simulink model "PID_dktocdo"  (Simulink 7.9)
settings: Solver=ode45  StartTime=0.0  StopTime=5  RelTol=1e-3
settings Model: Creator=Vaio  LastModifiedBy=Vaio

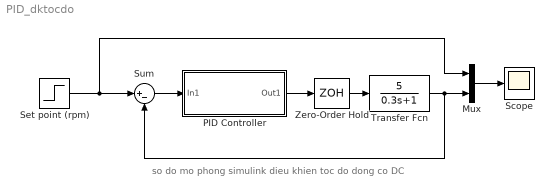
== system PID_dktocdo ==
  note: so do mo phong simulink dieu khien toc do dong co DC
  Mux : Mux  Inputs=2
  PID Controller : Subsystem
  Scope : Scope
  Set point (rpm) : Step  Time=0  After=800  SampleTime=0.005
  Sum : Sum  Inputs=|+-
  Transfer Fcn : TransferFcn  Numerator=[5]  Denominator=[0.3 1]
  Zero-Order Hold : ZeroOrderHold  SampleTime=0.005
  wires:
  Mux/1 -> Scope/1
  Transfer Fcn/1 -> Mux/2, Sum/2
  PID Controller/1(Out1) -> Zero-Order Hold/1
  Zero-Order Hold/1 -> Transfer Fcn/1
  Sum/1 -> PID Controller/1(In1)
  Set point (rpm)/1 -> Sum/1, Mux/1

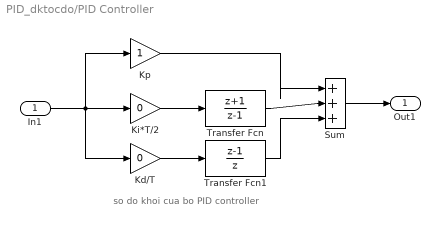
== system PID_dktocdo/PID Controller ==
  note: so do khoi cua bo PID controller
  In1 : Inport
  Kd/T : Gain  Gain=0  SampleTime=0.005
  Ki*T/2 : Gain  Gain=0  SampleTime=0.005
  Kp : Gain  SampleTime=0.005
  Sum : Sum  Inputs=|+++
  Transfer Fcn : DiscreteTransferFcn  Numerator=[1 1]  Denominator=[1 -1]  SampleTime=0.005
  Transfer Fcn1 : DiscreteTransferFcn  Numerator=[1 -1]  Denominator=[1 0]  SampleTime=0.005
  Out1 : Outport
  wires:
  In1/1 -> Kp/1, Ki*T/2/1, Kd/T/1
  Ki*T/2/1 -> Transfer Fcn/1
  Kd/T/1 -> Transfer Fcn1/1
  Transfer Fcn/1 -> Sum/2
  Sum/1 -> Out1/1
  Transfer Fcn1/1 -> Sum/3
  Kp/1 -> Sum/1
